simulink model "PX30eeees"  (R2015b)
settings: Solver=VariableStepAuto  StartTime=0.0  StopTime=5  RelTol=1e-3
settings Model: Creator=xmax1946  LastModifiedBy=xmax1946

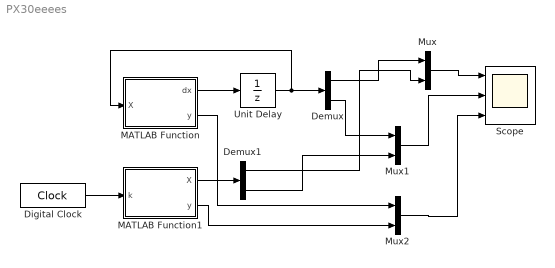
== system PX30eeees ==
  Demux : Demux  Outputs=2
  Demux1 : Demux  Outputs=2
  Digital Clock : DigitalClock
  MATLAB Function : MATLAB Function  TreatAsAtomicUnit=on
  MATLAB Function1 : MATLAB Function  TreatAsAtomicUnit=on
  Mux : Mux  Inputs=2
  Mux1 : Mux  Inputs=2
  Mux2 : Mux  Inputs=2
  Scope : Scope  NumInputPorts=3
  Unit Delay : UnitDelay  InitialCondition=[-1;-1]
  wires:
  MATLAB Function/1(dx) -> Unit Delay/1
  Unit Delay/1 -> Demux/1, MATLAB Function/1(X)
  Digital Clock/1 -> MATLAB Function1/1(k)
  Mux/1 -> Scope/1
  Mux1/1 -> Scope/2
  Mux2/1 -> Scope/3
  Demux/1 -> Mux/1
  MATLAB Function1/1(X) -> Demux1/1
  Demux1/1 -> Mux/2
  Demux/2 -> Mux1/1
  Demux1/2 -> Mux1/2
  MATLAB Function/2(y) -> Mux2/1
  MATLAB Function1/2(y) -> Mux2/2

== matlab function PX30eeees/MATLAB Function1 ==
  data: X output; k input; y output
function [X,y] = fcn(k)
C=[1,1];

X=[(85*(4/5)^k)/4 - (89*2^k)/4
             50 - 51*(4/5)^k];
y=C*X;

== matlab function PX30eeees/MATLAB Function ==
  data: dx output; X input; y output
function [dx,y]= fcn(X)
A=[2,.5;0,.8];
B=[-5;2];
C=[1,1];

dx=A*X+B*5;
y = C*X;
